simulink model "model_sim"  (R2016a)
settings: Solver=ode4  StartTime=0.0  StopTime=10.0  FixedStep=0.001  MaxStep=0.01  RelTol=1e-3
values from neighbouring files (symbols this model uses):
  Da = X0(5)    [cel.m]    (also in zad1.m)
  Dx = X0(3)    [cel.m]    (also in zad1.m)
  Ix = X0(2)    [cel.m]    (also in zad1.m)
  Km = 0.0265    [all2.m]    (also in cel.m; motor_x.m; motor_y.m)
  limit = 20    [dane.m]    (also in rk4.m; zad1.m)
  lin = 2    [all2.m]    (also in dane.m = 1; zad1.m = 10)
  mc = 1    [dane.m]    (also in obiekt.m; zad1.m)
  mw = X0    [celMW.m]    (also in dane.m = 1.155; obiekt.m = 1.155; zad1.m = 1.155)
  p = 60    [dane.m]    (also in zad1.m)
  Pa = X0(4)    [cel.m]    (also in zad1.m)
  Px = X0(1)    [cel.m]    (also in zad1.m)
  Rn = 0.0185    [dane.m]    (also in obiekt.m; zad1.m)
libraries: simulink x2
settings Model: Creator=Maciek  LastModifiedBy=Maciek

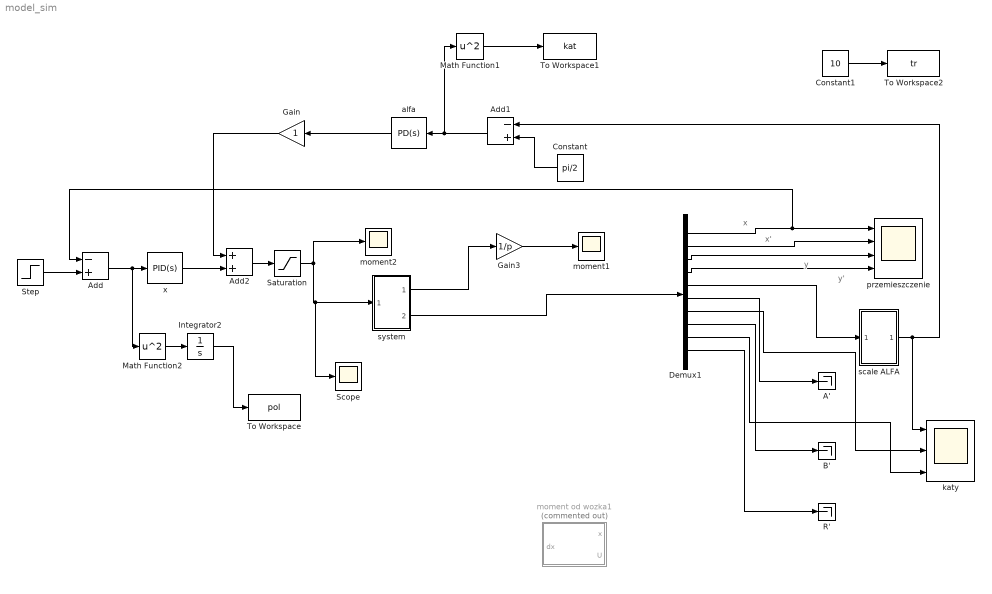
== system model_sim ==
  note: y'
  note: y
  note: x'
  note: x
  A' : Terminator
  Add : Sum  Inputs=-+
  Add1 : Sum  Inputs=-+
  Add2 : Sum
  B' : Terminator
  Constant : Constant  Value=pi/2
  Constant1 : Constant  Value=10
  Demux1 : Demux  Outputs=10
  Gain : Gain
  Gain3 : Gain  Gain=1/p
  Integrator2 : Integrator
  Math Function1 : Math  Operator=square  SaturateOnIntegerOverflow=on
  Math Function2 : Math  Operator=square  SaturateOnIntegerOverflow=on
  R' : Terminator
  Saturation : Saturate  UpperLimit=limit  LowerLimit=-limit
  Scope : Scope
  Step : Step  Time=0.1  After=0.2  SampleTime=0
  To Workspace : ToWorkspace  VariableName=pol  SampleTime=-1
      settings: MaxDataPoints=1
  To Workspace1 : ToWorkspace  VariableName=kat  SampleTime=-1
  To Workspace2 : ToWorkspace  VariableName=tr  SampleTime=-1
      settings: MaxDataPoints=1
  alfa : simulink/Continuous/PID Controller  Controller=PD  TimeDomain=Continuous-time  SampleTime=-1  IntegratorMethod=Forward Euler  FilterMethod=Forward Euler  Form=Parallel  UseFilter=on  ControllerParametersSource=internal  P=Pa  I=0.005  D=Da  N=100  InitialConditionSource=internal  InitialConditionForIntegrator=0  InitialConditionForFilter=0  ExternalReset=none  LimitOutput=on  UpperSaturationLimit=limit  LowerSaturationLimit=-limit  LinearizeAsGain=on  AntiWindupMode=none  Kb=1  TrackingMode=off  Kt=1  PParamMin=[]  PParamMax=[]  IParamMin=[]  IParamMax=[]  DParamMin=[]  DParamMax=[]  NParamMin=[]  NParamMax=[]  KbParamMin=[]  KbParamMax=[]  KtParamMin=[]  KtParamMax=[]  POutMin=[]  POutMax=[]  IOutMin=[]  IOutMax=[]  DOutMin=[]  DOutMax=[]  NOutMin=[]  NOutMax=[]  KbOutMin=[]  KbOutMax=[]  KtOutMin=[]  KtOutMax=[]  IntegratorOutMin=[]  IntegratorOutMax=[]  FilterOutMin=[]  FilterOutMax=[]  SumOutMin=[]  SumOutMax=[]  SumI1OutMin=[]  SumI1OutMax=[]  SumI2OutMin=[]  SumI2OutMax=[]  SumI3OutMin=[]  SumI3OutMax=[]  SumDOutMin=[]  SumDOutMax=[]  SaturationOutMin=[]  SaturationOutMax=[]  IntegratorContinuousStateAttributes=''  IntegratorStateMustResolveToSignalObject=off  IntegratorRTWStateStorageClass=Auto  FilterContinuousStateAttributes=''  FilterStateMustResolveToSignalObject=off  FilterRTWStateStorageClass=Auto  DifferentiatorICPrevScaledInput=0  DifferentiatorOutMin=[]  DifferentiatorOutMax=[]
  katy : Scope  NumInputPorts=3
  moment od wozka1 : MATLAB Function  Commented=on  TreatAsAtomicUnit=on
  moment1 : Scope
  moment2 : Scope
  przemieszczenie : Scope  NumInputPorts=4
  scale ALFA : Subsystem
  system : Subsystem
  x : simulink/Continuous/PID Controller  Controller=PID  TimeDomain=Continuous-time  SampleTime=-1  IntegratorMethod=Forward Euler  FilterMethod=Forward Euler  Form=Parallel  UseFilter=on  ControllerParametersSource=internal  P=Px  I=Ix  D=Dx  N=100  InitialConditionSource=internal  InitialConditionForIntegrator=0  InitialConditionForFilter=0  ExternalReset=none  LimitOutput=on  UpperSaturationLimit=limit  LowerSaturationLimit=-limit  LinearizeAsGain=on  AntiWindupMode=none  Kb=1  TrackingMode=off  Kt=1  PParamMin=[]  PParamMax=[]  IParamMin=[]  IParamMax=[]  DParamMin=[]  DParamMax=[]  NParamMin=[]  NParamMax=[]  KbParamMin=[]  KbParamMax=[]  KtParamMin=[]  KtParamMax=[]  POutMin=[]  POutMax=[]  IOutMin=[]  IOutMax=[]  DOutMin=[]  DOutMax=[]  NOutMin=[]  NOutMax=[]  KbOutMin=[]  KbOutMax=[]  KtOutMin=[]  KtOutMax=[]  IntegratorOutMin=[]  IntegratorOutMax=[]  FilterOutMin=[]  FilterOutMax=[]  SumOutMin=[]  SumOutMax=[]  SumI1OutMin=[]  SumI1OutMax=[]  SumI2OutMin=[]  SumI2OutMax=[]  SumI3OutMin=[]  SumI3OutMax=[]  SumDOutMin=[]  SumDOutMax=[]  SaturationOutMin=[]  SaturationOutMax=[]  IntegratorContinuousStateAttributes=''  IntegratorStateMustResolveToSignalObject=off  IntegratorRTWStateStorageClass=Auto  FilterContinuousStateAttributes=''  FilterStateMustResolveToSignalObject=off  FilterRTWStateStorageClass=Auto  DifferentiatorICPrevScaledInput=0  DifferentiatorOutMin=[]  DifferentiatorOutMax=[]
  wires:
  Demux1/10 -> R'/1
  Demux1/8 -> B'/1
  Demux1/7 -> katy/2
  Demux1/9 -> katy/3
  Demux1/6 -> A'/1
  Demux1/2 -> przemieszczenie/2
  Demux1/3 -> przemieszczenie/3
  Demux1/4 -> przemieszczenie/4
  Demux1/5 -> scale ALFA/1(In1)
  Demux1/1 -> Add/1, przemieszczenie/1
  Gain3/1 -> moment1/1
  system/1(Out1) -> Gain3/1
  system/2(Out2) -> Demux1/1
  Step/1 -> Add/2
  Constant/1 -> Add1/2
  x/1 -> Add2/2
  alfa/1 -> Gain/1
  Add2/1 -> Saturation/1
  Saturation/1 -> Scope/1, system/1(In1), moment2/1
  Gain/1 -> Add2/1
  scale ALFA/1(Out1) -> Add1/1, katy/1
  Add1/1 -> Math Function1/1, alfa/1
  Add/1 -> Math Function2/1, x/1
  Math Function2/1 -> Integrator2/1
  Math Function1/1 -> To Workspace1/1
  Integrator2/1 -> To Workspace/1
  Constant1/1 -> To Workspace2/1

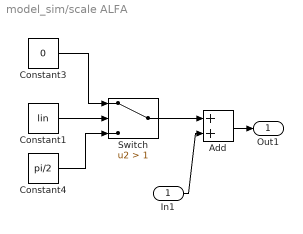
== system model_sim/scale ALFA ==
  In1 : Inport
  Add : Sum  Inputs=2
  Constant1 : Constant  Value=lin
  Constant3 : Constant  Value=0
  Constant4 : Constant  Value=pi/2
  Switch : Switch  Criteria=u2 > Threshold  Threshold=1
  Out1 : Outport
  wires:
  Add/1 -> Out1/1
  In1/1 -> Add/2
  Constant4/1 -> Switch/3
  Constant3/1 -> Switch/1
  Switch/1 -> Add/1
  Constant1/1 -> Switch/2

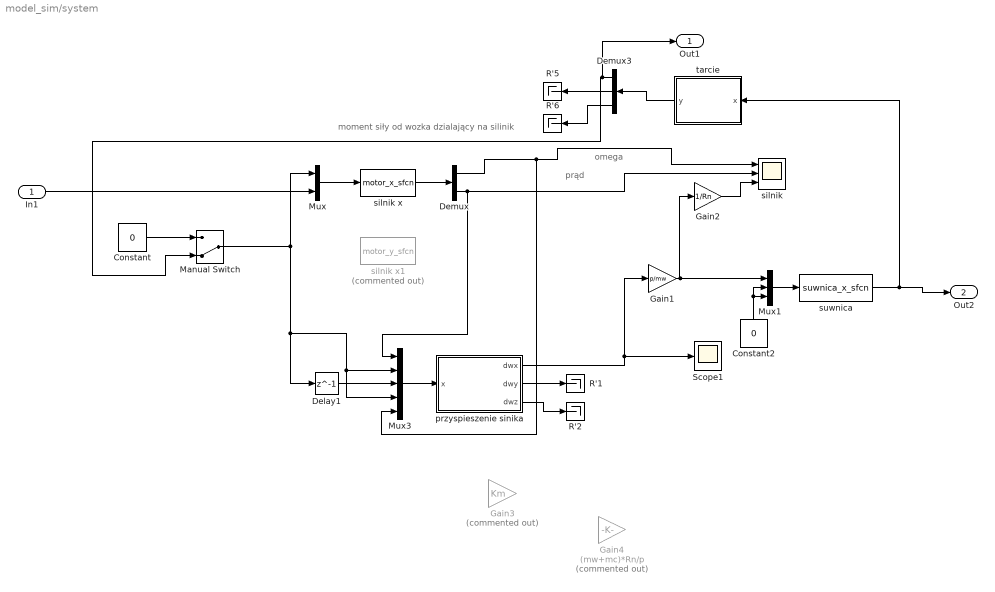
== system model_sim/system ==
  note: moment siły od wozka dzialający na silinik
  note: prąd
  note: omega
  In1 : Inport
  Constant : Constant  Value=0
  Constant2 : Constant  Value=0
  Delay1 : Delay  DelayLength=1
  Demux : Demux  Outputs=2
  Demux3 : Demux  Outputs=3
  Gain1 : Gain  Gain=p/mw
  Gain2 : Gain  Gain=1/Rn
  Gain3 : Gain  Commented=on  Gain=Km
  Gain4 : Gain  Commented=on  Gain=(mw+mc)*Rn/p
  Manual Switch : ManualSwitch  CurrentSetting=0
  Mux : Mux  Inputs=2
  Mux1 : Mux  Inputs=3
  Mux3 : Mux  Inputs=5
  R'{1..2,5..6} (4 alike) : Terminator
  Scope1 : Scope
  przyspieszenie sinika : MATLAB Function  TreatAsAtomicUnit=on
  silnik : Scope  NumInputPorts=3
  silnik x : S-Function  FunctionName=motor_x_sfcn  SFunctionDeploymentMode=off  EnableBusSupport=off
  silnik x1 : S-Function  Commented=on  FunctionName=motor_y_sfcn  SFunctionDeploymentMode=off  EnableBusSupport=off
  suwnica : S-Function  FunctionName=suwnica_x_sfcn  Parameters=x0  SFunctionDeploymentMode=off  EnableBusSupport=off
  tarcie : MATLAB Function  TreatAsAtomicUnit=on
  Out1 : Outport
  Out2 : Outport  Port=2
  wires:
  In1/1 -> Mux/2
  Mux/1 -> silnik x/1
  silnik x/1 -> Demux/1
  Mux1/1 -> suwnica/1
  Constant2/1 -> Mux1/2, Mux1/3
  Mux3/1 -> przyspieszenie sinika/1(x)
  przyspieszenie sinika/3(dwz) -> R'2/1
  przyspieszenie sinika/2(dwy) -> R'1/1
  suwnica/1 -> Out2/1, tarcie/1(x)
  Demux/2 -> Mux3/1, silnik/2
  Delay1/1 -> Mux3/3
  Constant/1 -> Manual Switch/1
  tarcie/1(y) -> Demux3/1
  Demux3/2 -> R'5/1
  Demux3/3 -> R'6/1
  Gain1/1 -> Mux1/1, Gain2/1
  Manual Switch/1 -> Mux/1, Delay1/1, Mux3/4, Mux3/2
  przyspieszenie sinika/1(dwx) -> Gain1/1, Scope1/1
  Demux3/1 -> Out1/1, Manual Switch/2
  Demux/1 -> Mux3/5, silnik/1
  Gain2/1 -> silnik/3

== matlab function model_sim/system/przyspieszenie sinika ==
  data: x input; dwx output; dwy output; dwz output
function [dwx, dwy, dwz] = angular_accel(x)

    %w = x(1); %predkosc katowa
    %temp = x(1);
    %ix = temp(2);
    wx = x(5);
    ix = x(1); % prad x
    iy = x(2); % prad x
    awx = x(3); %przysp x
    awy = x(4); %przys y
    
    xs = 1.5;   % szerokość suwnicy
    sy = 2.5;   % dł suwnicy
    mw = 1.155;%2.49;  % masa wózka
    ms = 2.2;%4.09;  % masa szyny
    mc = 1;     % masa ciężarka
    Rn = 0.0185;% promien bloków napedzajacych
    g = 9.81;
    p = 20;%przekladnia
    
    J = 1.1418*10^(-6);   %moment bezwladnisci
    tau_e = 0.48*10^(-3);
    tau_m = 21*10^(-3);                                                                             
    Ke = 0.02607;  %stala elektryczna
    Km = 0.0265;    %stala mechaniczna
    R = 12.5;      %opornosc
    L = 5.93*10^(-3);    %indukcyjnosc
    
    Mx = mw + mc;
    My = mw + ms + mc;
    
    dwx = (Km * ix - awx * Mx * Rn /p - 0* wx) ;%/ J;
    
    dwy = (Km * iy - awy * My * Rn / p ) ;%/ J;
    
    dwz = 0;%Km/J * i - aw * Mx * Rn / J;
    
end

== matlab function model_sim/system/tarcie ==
  data: x input; y output
function y  = tarcie(x)
%#codegen

    xs = 1.5;   % szerokość suwnicy
    sy = 2.5;   % dł suwnicy
    mw = 1.155;%2.49;  % masa wózka
    ms = 2.2;%4.09;  % masa szyny
    mc = 1;     % masa ciężarka
    Rn = 0.0185;% promien bloków napedzajacych
    g = 9.81;
    
    k1 = 82;%75;
    k2 = 100;%75;
    k3 = 75;%75;
    %siły tarcia
    if x(2) > 0 
        Tx = k1*mw*x(2) + 7.5;%10;
    elseif x(2) < 0
        Tx = k1*mw*x(2) - 7.5;%10;
    else
        Tx = 0;
    end
    if x(4) > 0 
        Ty = k2*(mw+ms)*x(4) + 5;%22;
    elseif x(4) < 0
        Ty = k2*(mw+ms)*x(4) - 5;%22;
    else
        Ty = 0;
    end
    if x(10) > 0
        Tr = -g*mc - x(10) * k3;%142;
    elseif x(10) < 0 
        Tr = g*mc - x(10) * k3;%218;
    else
        Tr = g*mc;
    end
    %Tr = k3*mc*x(10);
    
    T1 = Tx/mw;
    T2 = Ty/(mw+mc);
    T3 = Tr/mc;
    y = zeros(3,1);
    y(1) = T1;
    y(2) = T2;
    y(3) = T3;
end

== matlab function model_sim/moment od wozka1 ==
  data: x input; dx output; U input
function dx   = torque_x(x, U)

    lin = 1;
    xs = 1.5;   % szerokość suwnicy
    sy = 2.5;   % dł suwnicy
    mw = 1.155;%2.49;  % masa wózka
    ms = 2.2;%4.09;  % masa szyny
    mc = 1;     % masa ciężarka
    Rn = 0.0185;% promien bloków napedzajacych
    g = 9.81;
    
    %wsp tarcia
    k1 = 82;%75;
    k2 = 100;%75;
    k3 = 75;%75;
    %siły tarcia
    if x(2) > 0 
        Tx = k1*mw*x(2) + 7.5;%10;
    elseif x(2) < 0
        Tx = k1*mw*x(2) - 7.5;%10;
    else
        Tx = 0;
    end
    if x(4) > 0 
        Ty = k2*(mw+ms)*x(4) + 5;%22;
    elseif x(4) < 0
        Ty = k2*(mw+ms)*x(4) - 5;%22;
    else
        Ty = 0;
    end
    if x(10) > 0
        Tr = -g*mc - x(10) * k3;%142;
    elseif x(10) < 0 
        Tr = g*mc - x(10) * k3;%218;
    else
        Tr = 0;
    end
    %Tr = k3*mc*x(10);
    
    T1 = Tx/mw;
    T2 = Ty/(mw+mc);
    T3 = Tr/mc;
    
    %u = [x(11) x(12) x(13)];
    u = U * Rn; % przejscie z przyspieszenia katowego na liniowe
    N1 = u(1) - T1;
    N2 = u(2) - T2;
    N3 = u(3) - T3;
    
    ni1 = mc/mw;
    ni2 = mc/(mw + ms);
    
    if lin == 1%model liniowy
        dx= zeros(3,1);
        dx(1) = N1-ni1*x(5)*N3;                             %xw'
        dx(2) = N2+ni2*x(7)*N3;                             %yw'
        dx(3) = -N3 +g;                                    %R'
    
    else %model nieliniowy
        dx= zeros(3,1);
        
        V5 = cos(x(5))*sin(x(5))*(x(8))^2*x(9) - 2*x(10)*x(6) + g*cos(x(5))*cos(x(7));
        V6 = 2*x(8)*(cos(x(5))*x(6)*x(9) + sin(x(5))*x(10)) + g*sin(x(7));
        V7 = (sin(x(5)))^2*(x(8))^2*x(9) + g*sin(x(5))*cos(x(7)) + x(6)*x(6)*x(9);
        
        dx(1) = N1+ni1*cos(x(5))*N3;
        dx(2) = N2 + ni2*sin(x(7))*sin(x(5))*N3;
        dx(3) = -cos(x(5))*N1 - sin(x(5))*sin(x(7))*N2 -(1+ni1*(cos(x(5)))^2+ni2*(sin(x(5)))^2*(sin(x(7)))^2)*N3+V7;
     end
    
end
